simulink model "Lab3"  (R2023a)
settings: Solver=VariableStepAuto  StartTime=0.0  StopTime=10.0  RelTol=1e-3
undefined symbols (not defined in the file): QAM, qammod
libraries: commfilt2 x2, commchan3 x1, commrflib2 x1, dspsigops x1, dspstat3 x1, commsink2 x1, commrandsrc3 x1
settings Model: Creator=Дима  LastModifiedBy=Дима

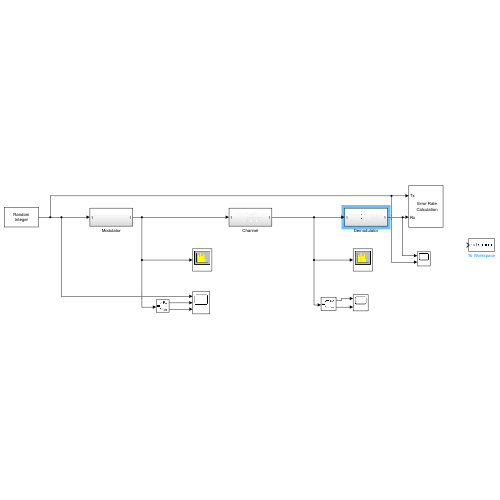
[thumbnail: Simulink's stored preview of the top-level diagram]
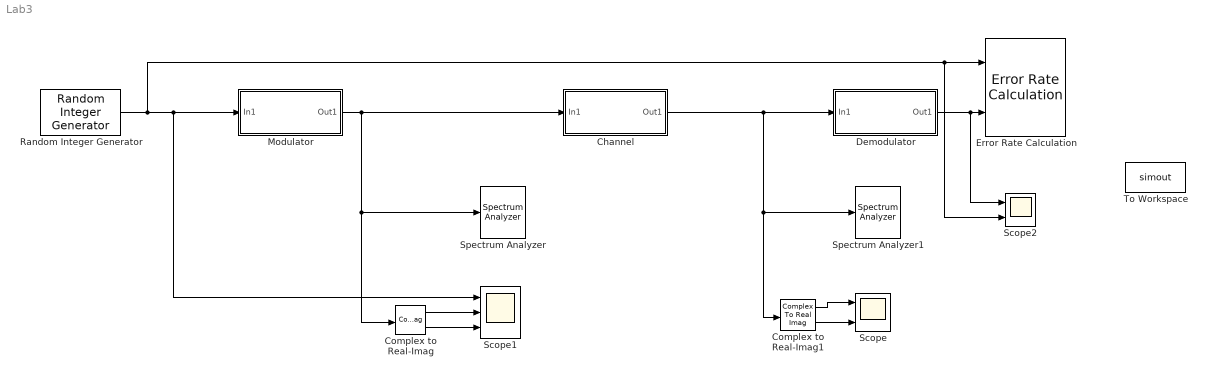
== system Lab3 ==
  Channel : Subsystem
  Complex to Real-Imag : ComplexToRealImag
  Complex to Real-Imag1 : ComplexToRealImag
  Demodulator : Subsystem
  Error Rate Calculation : commsink2/Error Rate Calculation  N=0  st_delay=0  cp_mode=Entire frame  subframe=[]  PMode=Workspace  WsName=ErrorVec  RsMode2=off  stop=off  numErr=100  maxBits=1e6
  Modulator : Subsystem
  Random Integer Generator : commrandsrc3/Random Integer Generator  SetSize=8  SeedSource=Auto  Seed=0  SampleTime=1  SamplesPerFrame=1  OutputDataType=double  SimulateUsing=Interpreted execution
  Scope : Scope  NumInputPorts=2
  Scope1 : Scope  NumInputPorts=3
  Scope2 : Scope  NumInputPorts=2
  Spectrum Analyzer : SpectrumAnalyzer  SampleRateSource=Property  SampleRate=44.1e3  PlotAsTwoSidedSpectrum=off  FrequencyScale=Log  FrequencySpan=Start and stop frequencies  StartFrequency=20  StopFrequency=20e3  YLimits=[-20 80]  ColorLimits=[-20 80]  DefaultConfigurationName=spbscopes.SpectrumAnalyzerBlockCfg  IsFrequencyInputMode=0  FrequencyVectorPort=0  FrequencyVectorFromPort=0  FrequencyInputRBWPort=0  FrequencyInputRBWFromPort=0
  Spectrum Analyzer1 : SpectrumAnalyzer  SampleRateSource=Property  SampleRate=44.1e3  PlotAsTwoSidedSpectrum=off  FrequencyScale=Log  FrequencySpan=Start and stop frequencies  StartFrequency=20  StopFrequency=20e3  YLimits=[-20 80]  ColorLimits=[-20 80]  DefaultConfigurationName=spbscopes.SpectrumAnalyzerBlockCfg  IsFrequencyInputMode=0  FrequencyVectorPort=0  FrequencyVectorFromPort=0  FrequencyInputRBWPort=0  FrequencyInputRBWFromPort=0
  To Workspace : ToWorkspace  VariableName=simout  SaveFormat=Timeseries  SampleTime=-1
  wires:
  Complex to Real-Imag1/2 -> Scope/2
  Complex to Real-Imag1/1 -> Scope/1
  Modulator/1(Out1) -> Channel/1(In1), Complex to Real-Imag/1, Spectrum Analyzer/1
  Random Integer Generator/1 -> Scope2/2, Error Rate Calculation/1, Modulator/1(In1), Scope1/1
  Complex to Real-Imag/2 -> Scope1/3
  Complex to Real-Imag/1 -> Scope1/2
  Channel/1(Out1) -> Demodulator/1(In1), Complex to Real-Imag1/1, Spectrum Analyzer1/1
  Demodulator/1(Out1) -> Scope2/1, Error Rate Calculation/2

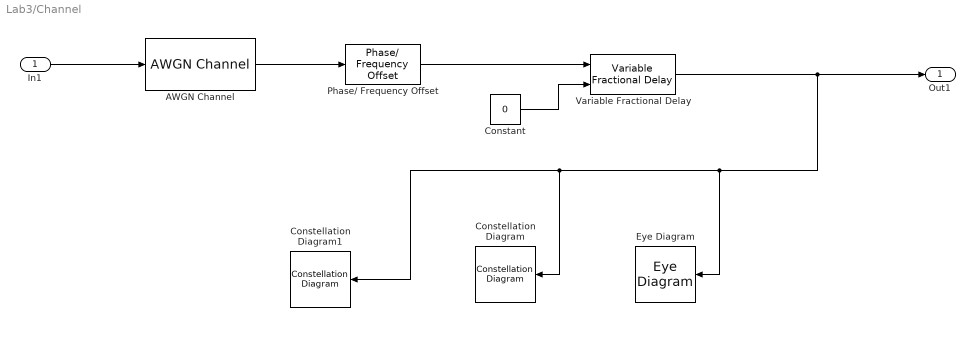
== system Lab3/Channel ==
  In1 : Inport
  AWGN Channel : commchan3/AWGN Channel  LegacyMode=off  NoiseMethod="Signal to noise ratio  (SNR)"  noiseMode="Signal to noise ratio  (SNR)"  EbNo=10  EsNo=10  SNR=13  BitsPerSymbol=1  SignalPower=1  SamplesPerSymbol=1  SymbolPeriod=1  VarianceSource=Parameter  Variance=1  RandomStream=Global stream  Seed=67  SimulateUsing=Code generation
  Constant : Constant  Value=0
  Constellation Diagram : ConstellationDiagram  WindowPosition=[139.000000,120.000000,600.000000,600.000000,]  ScopeFrameLocation=window  ShowTrajectory=on
  Constellation Diagram1 : ConstellationDiagram  WindowPosition=[382.000000,84.000000,600.000000,600.000000,]  ScopeFrameLocation=window  ReferenceConstellation=256-QAM
  Eye Diagram : EyeDiagram
  Phase/ Frequency Offset : commrflib2/Phase// Frequency Offset  phaseOffset=0  freqPort=off  freqOffset=0
  Variable Fractional Delay : dspsigops/Variable Fractional Delay  mode=OBSOLETE  modeActive=Linear  L=4  FarrowL=4  R=10  alpha=1  dmax=100  InputProcessing=Columns as channels (frame based)  ic=0  noDFT=off  fallbackFIR=Clip to the minimum value necessary for centered kernel  fallbackFarrow=Clip to the minimum value necessary for centered kernel  roundingMode=Zero  overflowMode=off
  Out1 : Outport
  wires:
  In1/1 -> AWGN Channel/1
  AWGN Channel/1 -> Phase/ Frequency Offset/1
  Phase/ Frequency Offset/1 -> Variable Fractional Delay/1
  Constant/1 -> Variable Fractional Delay/2
  Variable Fractional Delay/1 -> Constellation Diagram/1, Constellation Diagram1/1, Eye Diagram/1, Out1/1

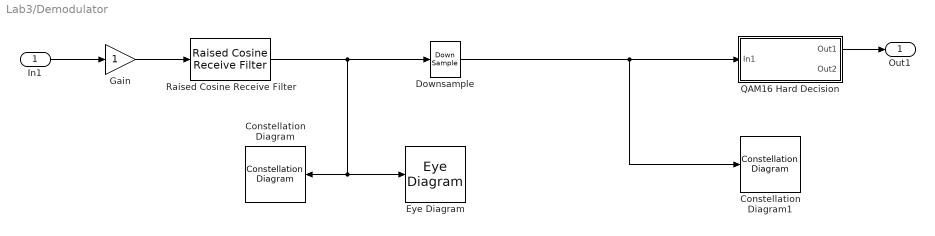
== system Lab3/Demodulator ==
  In1 : Inport
  Constellation Diagram : ConstellationDiagram
  Constellation Diagram1 : ConstellationDiagram
  Downsample : DownSample  N=8  RateOptions=Allow multirate processing
  Eye Diagram : EyeDiagram
  Gain : Gain
  QAM16 Hard Decision : Subsystem
  Raised Cosine Receive Filter : commfilt2/Raised Cosine Receive Filter  filtType=Square root  R=0.8  filtSpan=10  N=8  downFactor=8  downOffset=0  filterGain=1  RateOptions=Allow multirate processing  framing=Mute  checkCoeff=off  variableName=rcRxFilt  currentFiltSpan=10  D=5  inputOffset=0  sampMode=Mute  saveAsFlag=0  rateMode=Downsampling  checkGain=Normalized  launchFVT=on  roundingMode=Floor  overflowMode=off  coeffDataTypeStr=Inherit: Same word length as input  coeffMin=[]  coeffMax=[]  coeffLastDataTypeStr=Inherit: Same word length as input  accumDataTypeStr=Inherit: Same as product output  accumLastDataTypeStr=Inherit: Same as product output  outputDataTypeStr=Inherit: Same as accumulator  outputMin=[]  outputMax=[]  outputLastDataTypeStr=Inherit: Same as accumulator
  Out1 : Outport
  wires:
  In1/1 -> Gain/1
  Gain/1 -> Raised Cosine Receive Filter/1
  Raised Cosine Receive Filter/1 -> Constellation Diagram/1, Eye Diagram/1, Downsample/1
  Downsample/1 -> Constellation Diagram1/1, QAM16 Hard Decision/1(In1)
  QAM16 Hard Decision/1(Out1) -> Out1/1

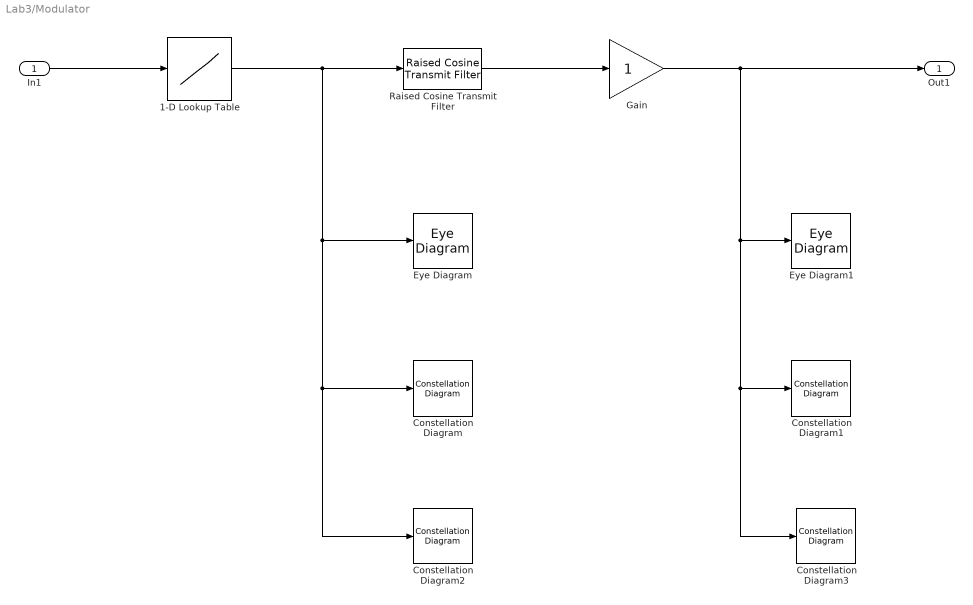
== system Lab3/Modulator ==
  In1 : Inport
  1-D Lookup Table : Lookup_n-D  NumberOfTableDimensions=1  BreakpointsForDimension1=[0:1:15]  Table=qammod([0:1:15],16)  InternalRulePriority=Speed  InputSameDT=off
  Constellation Diagram : ConstellationDiagram  WindowPosition=[512 294 341 345]  ScopeFrameLocation=window  SymbolsToDisplaySource=Property  SymbolsToDisplay=1000  ReferenceConstellation=16-QAM  XLimits=[-3.75 3.75]  YLimits=[-3.75 3.75]  ShowTrajectory=on  DefaultConfigurationName=comm.scopes.ConstellationDiagramBlockCfg
      settings: OpenAtSimulationStart=off
  Constellation Diagram1 : ConstellationDiagram  WindowPosition=[400 558 601 345]  ScopeFrameLocation=window  SymbolsToDisplaySource=Property  SymbolsToDisplay=1000  ReferenceConstellation=16-QAM  XLimits=[-1.9404 1.9409]  YLimits=[-1.9404 1.9409]  ShowTrajectory=on  EnableMeasurements=on  DefaultConfigurationName=comm.scopes.ConstellationDiagramBlockCfg
  Constellation Diagram2 : ConstellationDiagram  WindowPosition=[420 364 601 345]  ScopeFrameLocation=window  SymbolsToDisplaySource=Property  SymbolsToDisplay=1000  ReferenceConstellation=16-QAM  XLimits=[-3 3]  YLimits=[-3.75 3.75]  EnableMeasurements=on  DefaultConfigurationName=comm.scopes.ConstellationDiagramBlockCfg
      settings: OpenAtSimulationStart=off
  Constellation Diagram3 : ConstellationDiagram  WindowPosition=[1016 485 601 345]  ScopeFrameLocation=window  SymbolsToDisplaySource=Property  SymbolsToDisplay=1000  ReferenceConstellation=16-QAM  XLimits=[-1.9199 1.917]  YLimits=[-1.9199 1.917]  EnableMeasurements=on  DefaultConfigurationName=comm.scopes.ConstellationDiagramBlockCfg
      settings: OpenAtSimulationStart=off
  Eye Diagram : EyeDiagram
  Eye Diagram1 : EyeDiagram
  Gain : Gain
  Raised Cosine Transmit Filter : commfilt2/Raised Cosine Transmit Filter  filtType=Square root  R=0.8  filtSpan=10  N=8  filterGain=1  RateOptions=Allow multirate processing  framing=Mute  checkCoeff=off  variableName=rcTxFilt  checkGain=Normalized  sampMode=Mute  saveAsFlag=0  currentFiltSpan=10  D=(10)/2  launchFVT=on  roundingMode=Floor  overflowMode=off  coeffDataTypeStr=Inherit: Same word length as input  coeffMin=[]  coeffMax=[]  coeffLastDataTypeStr=Inherit: Same word length as input  outputDataTypeStr=Inherit: Same as accumulator  outputMin=[]  outputMax=[]  outputLastDataTypeStr=Inherit: Same as accumulator
  Out1 : Outport
  wires:
  Gain/1 -> Out1/1, Eye Diagram1/1, Constellation Diagram1/1, Constellation Diagram3/1
  In1/1 -> 1-D Lookup Table/1
  1-D Lookup Table/1 -> Raised Cosine Transmit Filter/1, Eye Diagram/1, Constellation Diagram/1, Constellation Diagram2/1
  Raised Cosine Transmit Filter/1 -> Gain/1

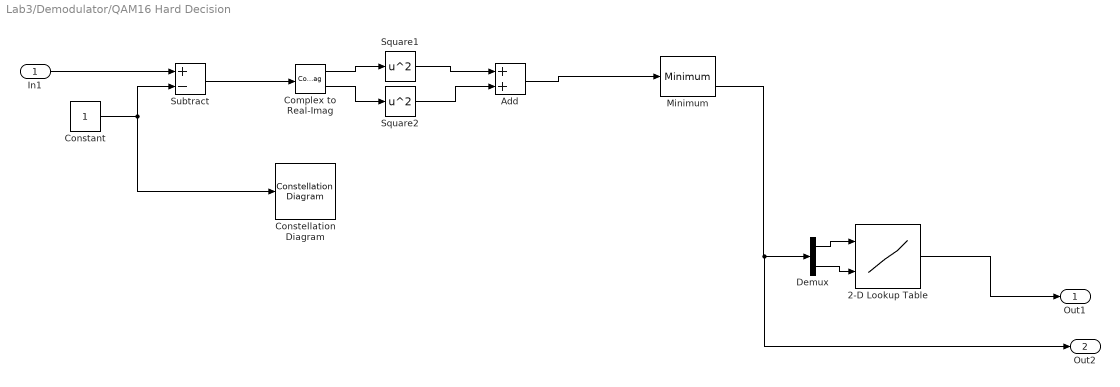
== system Lab3/Demodulator/QAM16 Hard Decision ==
  In1 : Inport
  2-D Lookup Table : Lookup_n-D  BreakpointsForDimension1=[1:3]  BreakpointsForDimension2=[1:3]  InternalRulePriority=Speed  RndMeth=Simplest
      settings: InputPortMap=u0,u1
  Add : Sum
  Complex to Real-Imag : ComplexToRealImag
  Constant : Constant
  Constellation Diagram : ConstellationDiagram  WindowPosition=[382.000000,84.000000,600.000000,600.000000,]  ScopeFrameLocation=window  DefaultConfigurationName=comm.scopes.ConstellationDiagramBlockCfg
  Demux : Demux  Outputs=2
  Minimum : dspstat3/Minimum  operation=minimum  fcn=Value and Index  indexBase=One  operateOver=Each column  Dimension=1  InputProcessing=Columns as channels (frame based)  reset=None  roiEnable=off  roiType=Rectangles  roiPortion=Entire ROI  roiOutput=Individual statistics for each ROI  roiFlag=off  roundingMode=Floor  overflowMode=off
      settings: LibrarySourceBlock=dsphdlsupportstat/Minimum
  Square1 : Math  Operator=square  OutputSignalType=real
  Square2 : Math  Operator=square  OutputSignalType=complex
      settings: LockScale=on
  Subtract : Sum  Inputs=+-
  Out1 : Outport
  Out2 : Outport  Port=2
  wires:
  In1/1 -> Subtract/1
  Constant/1 -> Constellation Diagram/1, Subtract/2
  Subtract/1 -> Complex to Real-Imag/1
  Complex to Real-Imag/2 -> Square2/1
  Complex to Real-Imag/1 -> Square1/1
  Square1/1 -> Add/1
  Square2/1 -> Add/2
  Add/1 -> Minimum/1
  Demux/1 -> 2-D Lookup Table/1
  Demux/2 -> 2-D Lookup Table/2
  Minimum/2 -> Out2/1, Demux/1
  2-D Lookup Table/1 -> Out1/1
